simulink model "power_gui"  (Simulink 6.0)
settings: Solver=ode15s  SolverMode=SingleTasking  StartTime=0.0  StopTime=0.05  RelTol=1e-4
libraries: powerlib x27
settings Model: Creator=patrice  LastModifiedBy=batserve  ExtModeTrigMode=oneshot  ExtModeArmWhenConnect=off  ExtModeAutoUpdateStatusClock=off
settings DataIOCC: ExternalInput=[]  LimitDataPoints=off  SaveOutput=off  SignalLoggingName=sigsOut
settings OptimizationCC: BlockReduction=off  BooleanDataType=off
settings DebuggingCC: AlgebraicLoopMsg=none  SolverPrmCheckMsg=none  UnconnectedLineMsg=none
settings HardwareCC: TargetUnknown=on
settings RTWCC: TemplateMakefile=grt_unix.tmf

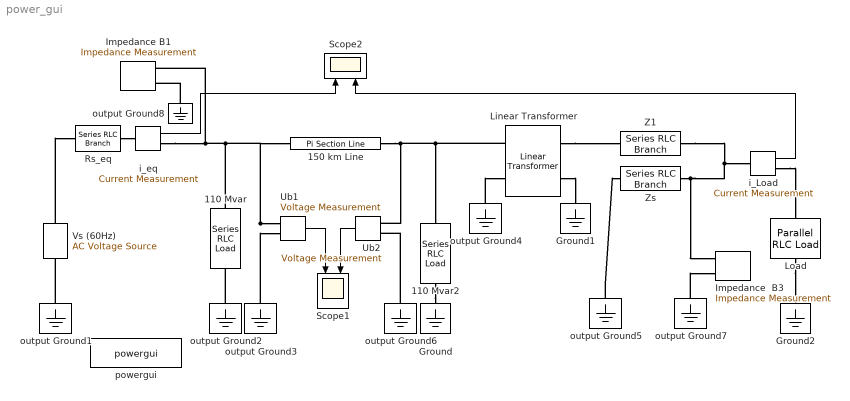
== system power_gui ==
  110 Mvar : powerlib/Elements/Series RLC Load  Orientation=up  PhysicalDomain=powersysdomain  SubClassName=unknown  LeftPortType=p1  RightPortType=p1  LConnTagsString=a  RConnTagsString=__new0  NominalVoltage=735000/sqrt(3)  NominalFrequency=60  ActivePower=110e6/300  InductivePower=110e6  CapacitivePower=0  Measurements=None
  110 Mvar2 : powerlib/Elements/Series RLC Load  Orientation=down  PhysicalDomain=powersysdomain  SubClassName=unknown  LeftPortType=p1  RightPortType=p1  LConnTagsString=a  RConnTagsString=__new0  NominalVoltage=735000/sqrt(3)  NominalFrequency=60  ActivePower=110e6/300  InductivePower=110e6  CapacitivePower=0  Measurements=None
  150 km Line : powerlib/Elements/Pi Section Line  PhysicalDomain=powersysdomain  SubClassName=unknown  LeftPortType=p1  RightPortType=p1  LConnTagsString=__new0  RConnTagsString=__new0  Frequency=60  Resistance=0.011  Inductance=0.8674e-03  Capacitance=13.41e-09  Length=150  PiSections=2  Measurements=None
      settings: AttributesFormatString=\n
  Ground : powerlib/Elements/Ground  Orientation=down  PhysicalDomain=powersysdomain  SubClassName=unknown  LeftPortType=p1  RightPortType=p1  LConnTagsString=a
  Ground1 : powerlib/Elements/Ground  Orientation=down  PhysicalDomain=powersysdomain  SubClassName=unknown  LeftPortType=p1  RightPortType=p1  LConnTagsString=a
  Ground2 : powerlib/Elements/Ground  Orientation=down  PhysicalDomain=powersysdomain  SubClassName=unknown  LeftPortType=p1  RightPortType=p1  LConnTagsString=a
  Impedance  B3 : powerlib/Measurements/Impedance Measurement  PhysicalDomain=powersysdomain  SubClassName=unknown  LeftPortType=p1  RightPortType=p1  LConnTagsString=+|-  Factor=1
      settings: AttributesFormatString=\n
  Impedance B1 : powerlib/Measurements/Impedance Measurement  Orientation=left  PhysicalDomain=powersysdomain  SubClassName=unknown  LeftPortType=p1  RightPortType=p1  LConnTagsString=+|-  Factor=1
      settings: AttributesFormatString=\n
  Linear Transformer : powerlib/Elements/Linear Transformer  PhysicalDomain=powersysdomain  SubClassName=unknown  LeftPortType=p1  RightPortType=p1  LConnTagsString=a|b  RConnTagsString=A|B  NominalPower=[750e6/3,60]  winding1=[735000/sqrt(3), 0.001 ,0.15]  winding2=[315000/sqrt(3), 0.001,0]  ThreeWindings=off  winding3=[315000/sqrt(3), 0.001,0]  RmLm=[500 500]  Measurements=None
  Load : powerlib/Elements/Parallel RLC Load  Orientation=down  PhysicalDomain=powersysdomain  SubClassName=unknown  LeftPortType=p1  RightPortType=p1  LConnTagsString=a  RConnTagsString=__new0  NominalVoltage=315000/sqrt(3)  NominalFrequency=60  ActivePower=200e6  InductivePower=0  CapacitivePower=50e6  Measurements=None
      settings: AttributesFormatString=\n
  Rs_eq : powerlib/Elements/Series RLC Branch  PhysicalDomain=powersysdomain  SubClassName=unknown  LeftPortType=p1  RightPortType=p1  LConnTagsString=__new0  RConnTagsString=__new0  Resistance=2  Inductance=0  Capacitance=inf  Measurements=None
  Scope1 : Scope  NumInputPorts=2
      settings: Orientation=down  TimeRange=0.05  YMin=-1e+006~-1e+006  YMax=1e+006~1e+006
  Scope2 : Scope  NumInputPorts=2
      settings: Orientation=up  TimeRange=0.05  YMin=-1000~-2000  YMax=3000~2000
  Ub1 : powerlib/Measurements/Voltage Measurement  Tag=PoWeRsYsTeMmEaSuReMeNt  PhasorSimulation=off  OutputType=Magnitude  PSBequivalent=0
  Ub2 : powerlib/Measurements/Voltage Measurement  Tag=PoWeRsYsTeMmEaSuReMeNt  Orientation=left  PhasorSimulation=off  OutputType=Magnitude  PSBequivalent=0
  Vs (60Hz) : powerlib/Electrical Sources/AC Voltage Source  Description=source block  Orientation=up  Amplitude=735000/sqrt(3)*sqrt(2)  Phase=0  Frequency=60  SampleTime=0  Measurements=None
      settings: AttributesFormatString=\n
  Z1 : powerlib/Elements/Series RLC Branch  PhysicalDomain=powersysdomain  SubClassName=unknown  LeftPortType=p1  RightPortType=p1  LConnTagsString=__new0  RConnTagsString=__new0  Resistance=0.734  Inductance=0.02085  Capacitance=inf  Measurements=None
  Zs : powerlib/Elements/Series RLC Branch  PhysicalDomain=powersysdomain  SubClassName=unknown  LeftPortType=p1  RightPortType=p1  LConnTagsString=__new0  RConnTagsString=__new0  Resistance=11.0  Inductance=0.2925  Capacitance=inf  Measurements=None
  i_Load : powerlib/Measurements/Current Measurement  Tag=PoWeRsYsTeMmEaSuReMeNt  PhasorSimulation=off  OutputType=Magnitude  PSBequivalent=0
  i_eq : powerlib/Measurements/Current Measurement  Tag=PoWeRsYsTeMmEaSuReMeNt  PhasorSimulation=off  OutputType=Magnitude  PSBequivalent=0
  output Ground{1..8} (8 alike) : powerlib/Elements/Ground  Orientation=down  PhysicalDomain=powersysdomain  SubClassName=unknown  LeftPortType=p1  RightPortType=p1  LConnTagsString=a
  powergui : powerlib/powergui  Priority=2  Frange=logspace(0,3,50)  Ylog=off  Xlog=off  save=off  variable=ZData  ZoomFFT=on  StartTime=0.0  cycles=2  DisplayStyle=off  fundamental=60  FreqAxis=off  MaxFrequency=1000  frequencyindice=1  frequencyindicesteady=1  RmsSteady=1  display=off  Ts=0  methode=off  frequency=60  echomessages=off
  wires:
  i_eq/1 -> Scope2/1
  Ub1/1 -> Scope1/1
  Ub2/1 -> Scope1/2
  i_Load/1 -> Scope2/2
  connections:
  output Ground1/LConn1 -- Vs (60Hz)/LConn1
  Vs (60Hz)/RConn1 -- Rs_eq/LConn1
  output Ground2/LConn1 -- 110 Mvar/LConn1
  Rs_eq/RConn1 -- i_eq/LConn1
  110 Mvar2/RConn1 -- Ground/LConn1
  output Ground3/LConn1 -- Ub1/LConn2
  Linear Transformer/LConn1 -- 150 km Line/RConn1 -- Ub2/LConn1 -- 110 Mvar2/LConn1
  output Ground6/LConn1 -- Ub2/LConn2
  Linear Transformer/RConn2 -- Ground1/LConn1
  output Ground4/LConn1 -- Linear Transformer/LConn2
  Zs/RConn1 -- Impedance  B3/LConn1 -- Z1/RConn1 -- i_Load/LConn1
  Load/RConn1 -- Ground2/LConn1
  i_Load/RConn1 -- Load/LConn1
  output Ground5/LConn1 -- Zs/LConn1
  Linear Transformer/RConn1 -- Z1/LConn1
  output Ground7/LConn1 -- Impedance  B3/LConn2
  150 km Line/LConn1 -- Ub1/LConn1 -- i_eq/RConn1 -- Impedance B1/LConn1 -- 110 Mvar/RConn1
  output Ground8/LConn1 -- Impedance B1/LConn2
